simulink model "Lab2_1_6"  (R2021b)
settings: Solver=VariableStepAuto  StartTime=0.0  StopTime=20  RelTol=1e-3
undefined symbols (not defined in the file): a, c, d
settings Model: Creator=george.tudor1906  LastModifiedBy=george.tudor1906

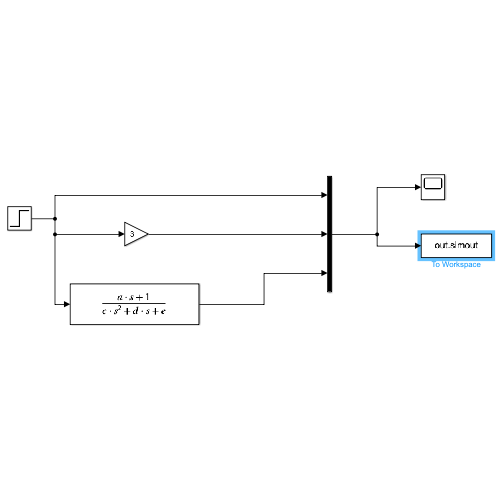
[thumbnail: Simulink's stored preview of the top-level diagram]
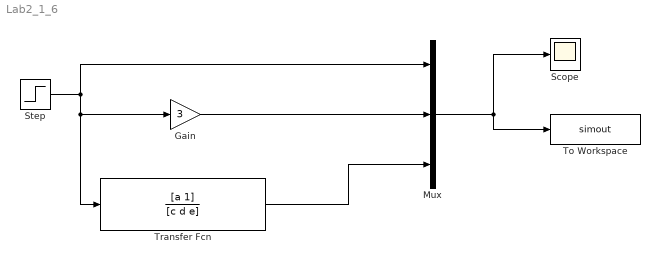
== system Lab2_1_6 ==
  Gain : Gain  Gain=3
  Mux : Mux  Inputs=3
  Scope : Scope
  Step : Step  Time=5  Before=2  After=4  SampleTime=0
  To Workspace : ToWorkspace  VariableName=simout  SaveFormat=Timeseries  SampleTime=-1
  Transfer Fcn : TransferFcn  Numerator=[a 1]  Denominator=[c d e]
  wires:
  Step/1 -> Gain/1, Transfer Fcn/1, Mux/1
  Gain/1 -> Mux/2
  Transfer Fcn/1 -> Mux/3
  Mux/1 -> To Workspace/1, Scope/1
